simulink model "debug_xSensIMU_legacy"  (Simulink 8.3)
settings: Solver=FixedStepDiscrete  StartTime=0.0  StopTime=inf  FixedStep=0.01  RelTol=1e-3
InitFcn:
  | ROBOT_DOF=23;
libraries: WBToolboxLibrary x7
settings Model: Creator=DanielePucci  LastModifiedBy=gnava  CovSFcnEnable=on
settings DataIOCC: SaveFormat=StructureWithTime  SignalLoggingSaveFormat=Dataset
settings DebuggingCC: UnderspecifiedInitializationDetection=Simplified  MergeDetectMultiDrivingBlocksExec=error  SolverPrmCheckMsg=none  FrameProcessingCompatibilityMsg=error  StateNameClashWarn=none
settings HardwareCC: ProdBitPerPointer=64  ProdLargestAtomicFloat=Float  ProdIntDivRoundTo=Zero  ProdEndianess=LittleEndian  ProdHWDeviceType=Specified
settings GRTTargetCC: GeneratePreprocessorConditionals=Use local settings  CombineOutputUpdateFcns=on  GRTInterface=off

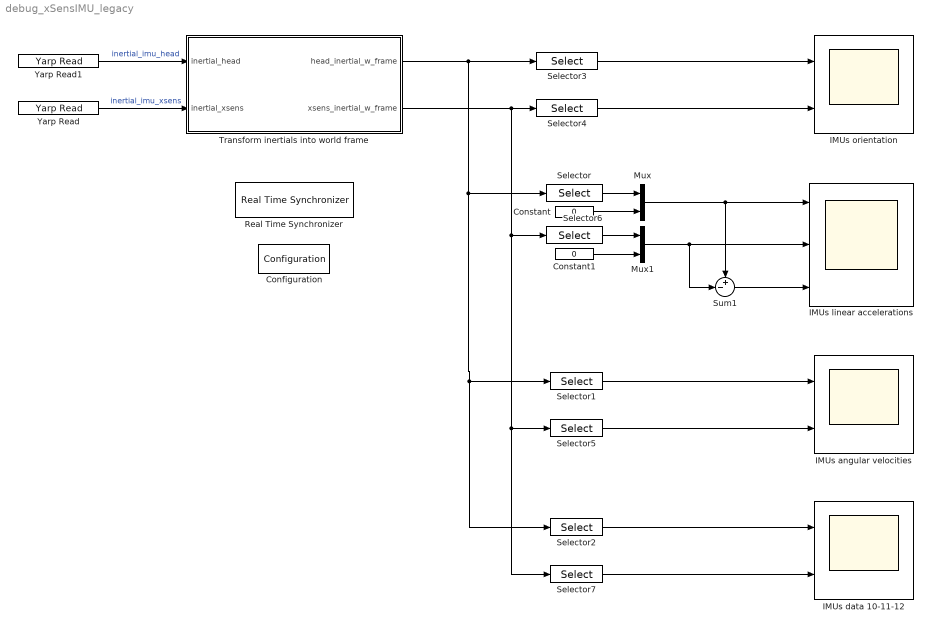
== system debug_xSensIMU_legacy ==
  Configuration : WBToolboxLibrary/Utilities/Configuration  ConfigSource=Workspace  ConfigObject='WBTConfigRobot'  RobotName='icub'  UrdfFile='model.urdf'  ControlledJoints={'l_elbow','l_shoulder_pitch','torso_roll'}  ControlBoardsNames={'left_arm','right_arm','torso'}  LocalName='WBT'  GravityVector=[0,0,-9.81]
  Constant : Constant  Value=0
  Constant1 : Constant  Value=0
  IMUs angular velocities : Scope  NumInputPorts=2
      settings: TimeRange=auto  ShowLegends=on  MaxDataPoints=5000  SaveToWorkspace=off  SaveName=ScopeData2  YMin=-37.69569~-33.78282  YMax=38.70376~30.66384  SampleTime=-1
  IMUs data 10-11-12 : Scope  NumInputPorts=2
      settings: TimeRange=auto  ShowLegends=on  MaxDataPoints=5000  SaveToWorkspace=off  SaveName=ScopeData3  YMin=-269.32411~-1.2142  YMax=88.18615~0.56889  SampleTime=-1
  IMUs linear accelerations : Scope  NumInputPorts=3
      settings: TimeRange=auto  ShowLegends=on  MaxDataPoints=5000  SaveToWorkspace=off  YMin=-5.95919~-4.60026~-4.97519  YMax=13.15614~13.38285~4.95253  SampleTime=-1
  IMUs orientation : Scope  NumInputPorts=2
      settings: TimeRange=auto  ShowLegends=on  MaxDataPoints=5000  SaveToWorkspace=off  SaveName=ScopeData3  YMin=-12.17243~-29.72159  YMax=49.15977~137.2842  SampleTime=-1
  Mux : Mux  Inputs=2
  Mux1 : Mux  Inputs=2
  Real Time Synchronizer : WBToolboxLibrary/Utilities/Real Time Synchronizer  period=0.01
  Selector : Selector  InputPortWidth=12  IndexOptions=Index vector (dialog)  Indices=[4:6]  OutputSizes=1
  Selector1 : Selector  InputPortWidth=12  IndexOptions=Index vector (dialog)  Indices=[7:9]  OutputSizes=1
  Selector2 : Selector  InputPortWidth=12  IndexOptions=Index vector (dialog)  Indices=[10:12]  OutputSizes=1
  Selector3 : Selector  InputPortWidth=12  IndexOptions=Index vector (dialog)  Indices=[1:3]  OutputSizes=1
  Selector4 : Selector  InputPortWidth=12  IndexOptions=Index vector (dialog)  Indices=[1:3]  OutputSizes=1
  Selector5 : Selector  InputPortWidth=12  IndexOptions=Index vector (dialog)  Indices=[7:9]  OutputSizes=1
  Selector6 : Selector  InputPortWidth=12  IndexOptions=Index vector (dialog)  Indices=[4:6]  OutputSizes=1
  Selector7 : Selector  InputPortWidth=12  IndexOptions=Index vector (dialog)  Indices=[10:12]  OutputSizes=1
  Sum1 : Sum  Inputs=+-|
  Transform inertials into world frame : Subsystem
  Yarp Read : WBToolboxLibrary/Utilities/Yarp Read  portName='/icub/xsens_inertial'  signalSize=12  timeout=0.5  blocking=off  timestamp=off  autoconnect=on  errorOnConnection=off
  Yarp Read1 : WBToolboxLibrary/Utilities/Yarp Read  portName='/icub/inertial'  signalSize=12  timeout=0.5  blocking=off  timestamp=off  autoconnect=on  errorOnConnection=off
  wires:
  Constant/1 -> Mux/2
  Selector1/1 -> IMUs angular velocities/1
  Selector2/1 -> IMUs data 10-11-12/1
  Selector3/1 -> IMUs orientation/1
  Yarp Read1/1 -> Transform inertials into world frame/1(inertial_head)  "inertial_imu_head"
  Yarp Read/1 -> Transform inertials into world frame/2(inertial_xsens)  "inertial_imu_xsens"
  Selector4/1 -> IMUs orientation/2
  Selector/1 -> Mux/1
  Constant1/1 -> Mux1/2
  Selector6/1 -> Mux1/1
  Mux/1 -> Sum1/1, IMUs linear accelerations/1
  Mux1/1 -> Sum1/2, IMUs linear accelerations/2
  Selector5/1 -> IMUs angular velocities/2
  Selector7/1 -> IMUs data 10-11-12/2
  Sum1/1 -> IMUs linear accelerations/3
  Transform inertials into world frame/1(head_inertial_w_frame) -> Selector2/1, Selector1/1, Selector/1, Selector3/1
  Transform inertials into world frame/2(xsens_inertial_w_frame) -> Selector7/1, Selector5/1, Selector6/1, Selector4/1

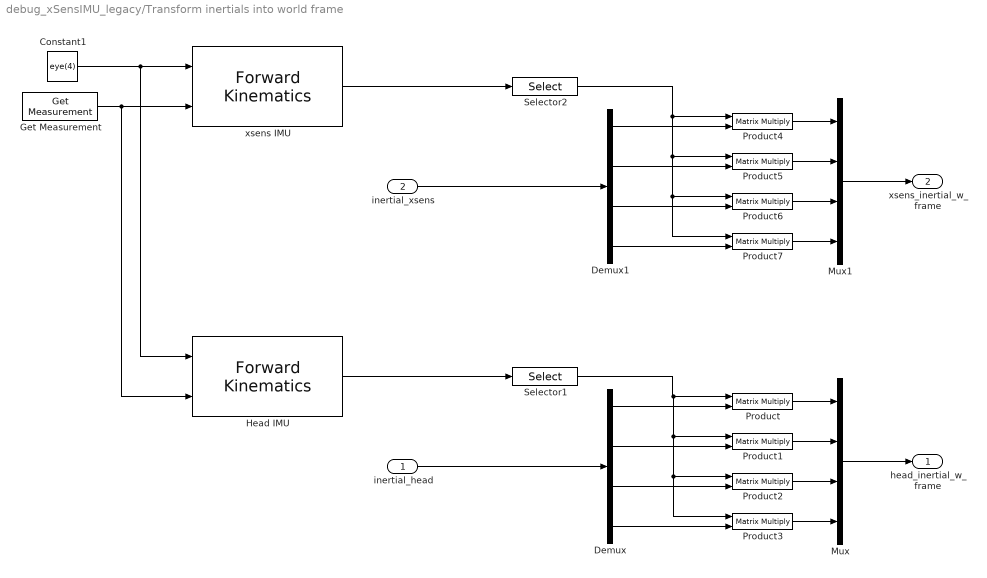
== system debug_xSensIMU_legacy/Transform inertials into world frame ==
  inertial_head : Inport
  inertial_xsens : Inport  Port=2
  Constant1 : Constant  Value=eye(4)
  Demux : Demux  Outputs=[3;3;3;3]
  Demux1 : Demux  Outputs=[3;3;3;3]
  Get Measurement : WBToolboxLibrary/wholeBodyStates/Get Measurement  measuredType=Joints Position
  Head IMU : WBToolboxLibrary/wholeBodyModel/Kinematics/Forward Kinematics  frameName='imu_frame'
  Mux : Mux
  Mux1 : Mux
  Product{,1..7} (8 alike) : Product  Multiplication=Matrix(*)
  Selector1 : Selector  NumberOfDimensions=2  InputPortWidth=12  IndexOptions=Index vector (dialog),Index vector (dialog)  Indices=[1:3],[1:3]  OutputSizes=1,1
  Selector2 : Selector  NumberOfDimensions=2  InputPortWidth=12  IndexOptions=Index vector (dialog),Index vector (dialog)  Indices=[1:3],[1:3]  OutputSizes=1,1
  xsens IMU : WBToolboxLibrary/wholeBodyModel/Kinematics/Forward Kinematics  frameName='root_link_imu_frame'
  head_inertial_w_frame : Outport
  xsens_inertial_w_frame : Outport  Port=2
  wires:
  Get Measurement/1 -> Head IMU/2, xsens IMU/2
  Constant1/1 -> Head IMU/1, xsens IMU/1
  Demux/1 -> Product/2
  Demux/3 -> Product2/2
  Demux/4 -> Product3/2
  Product/1 -> Mux/1
  Product1/1 -> Mux/2
  Product2/1 -> Mux/3
  Product3/1 -> Mux/4
  Demux/2 -> Product1/2
  Mux/1 -> head_inertial_w_frame/1
  Product6/1 -> Mux1/3
  Product5/1 -> Mux1/2
  Demux1/4 -> Product7/2
  Product7/1 -> Mux1/4
  Demux1/2 -> Product5/2
  Demux1/3 -> Product6/2
  Mux1/1 -> xsens_inertial_w_frame/1
  Demux1/1 -> Product4/2
  inertial_head/1 -> Demux/1
  Head IMU/1 -> Selector1/1
  xsens IMU/1 -> Selector2/1
  Product4/1 -> Mux1/1
  inertial_xsens/1 -> Demux1/1
  Selector1/1 -> Product3/1, Product2/1, Product1/1, Product/1
  Selector2/1 -> Product6/1, Product7/1, Product5/1, Product4/1
